simulink model "imfSILClaws"  (R2019a)
settings: Solver=FixedStepAuto  StartTime=0.0  StopTime=inf  FixedStep=.0125  RelTol=1e-3
libraries: etargetslib x2, dspnetwork x2, sldrtlib x1
settings Model: Creator=Chris  LastModifiedBy=Chris

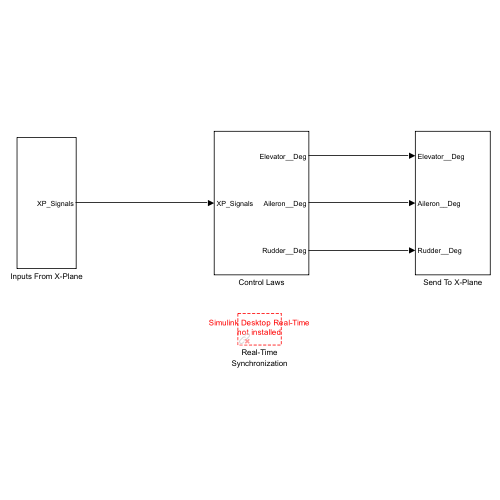
[thumbnail: Simulink's stored preview of the top-level diagram]
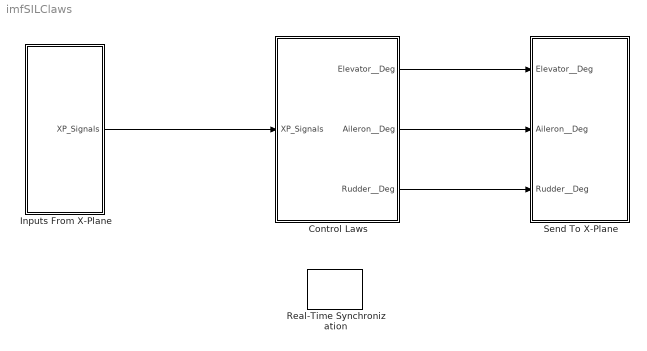
== system imfSILClaws ==
  Control Laws : Subsystem
  Inputs From X-Plane : Subsystem
  Real-Time Synchronization : sldrtlib/Real-Time Synchronization  SampleTime=.0125  MaxMissedTicks=10  ShowMissedTicks=off  YieldWhenWaiting=off
  Send To X-Plane : Subsystem
  wires:
  Inputs From X-Plane/1(XP_Signals) -> Control Laws/1(XP_Signals)
  Control Laws/1(Elevator__Deg) -> Send To X-Plane/1(Elevator__Deg)
  Control Laws/2(Aileron__Deg) -> Send To X-Plane/2(Aileron__Deg)
  Control Laws/3(Rudder__Deg) -> Send To X-Plane/3(Rudder__Deg)

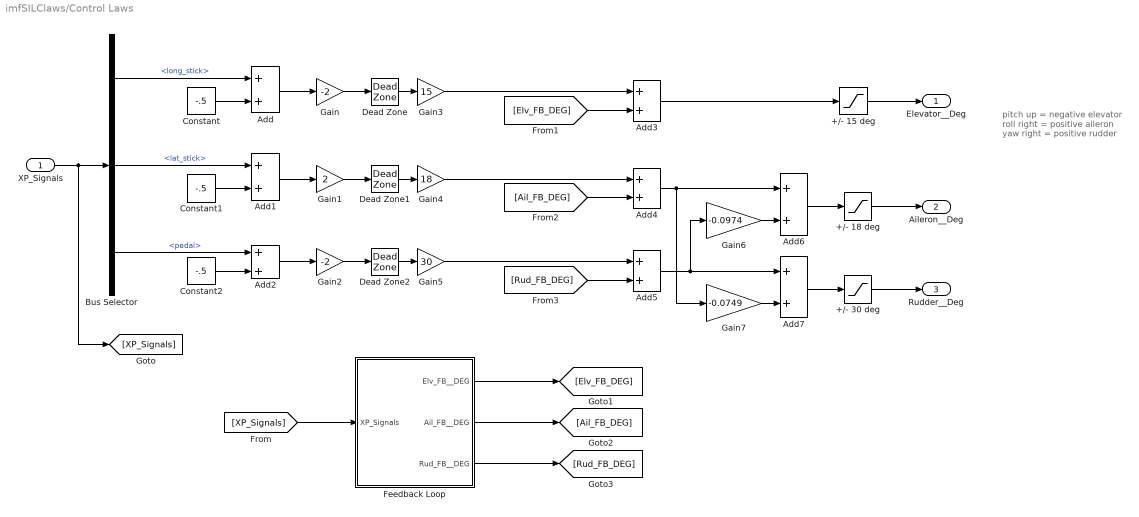
== system imfSILClaws/Control Laws ==
  note: pitch up = negative elevator
      | roll right = positive aileron
      | yaw right = positive rudder
  XP_Signals : Inport
  +/- 15 deg : Saturate  UpperLimit=15  LowerLimit=-15
  +/- 18 deg : Saturate  UpperLimit=18  LowerLimit=-18
  +/- 30 deg : Saturate  UpperLimit=30  LowerLimit=-30
  Add{,1..7} (8 alike) : Sum
  Bus Selector : BusSelector  OutputSignals=long_stick,lat_stick,pedal
  Constant : Constant  Value=-.5  OutDataTypeStr=single
  Constant1 : Constant  Value=-.5  OutDataTypeStr=single
  Constant2 : Constant  Value=-.5  OutDataTypeStr=single
  Dead Zone : DeadZone  LowerValue=-0.05  UpperValue=0.05  SaturateOnIntegerOverflow=on
  Dead Zone1 : DeadZone  LowerValue=-0.05  UpperValue=0.05  SaturateOnIntegerOverflow=on
  Dead Zone2 : DeadZone  LowerValue=-0.05  UpperValue=0.05  SaturateOnIntegerOverflow=on
  Feedback Loop : Subsystem
  Gain : Gain  Gain=-2
  Gain1 : Gain  Gain=2
  Gain2 : Gain  Gain=-2
  Gain3 : Gain  Gain=15
  Gain4 : Gain  Gain=18
  Gain5 : Gain  Gain=30
  Gain6 : Gain  Gain=-0.0974
  Gain7 : Gain  Gain=-0.0749
  Elevator__Deg : Outport
  Aileron__Deg : Outport  Port=2
  Rudder__Deg : Outport  Port=3
  wires:
  XP_Signals/1 -> [XP_Signals], Bus Selector/1
  +/- 18 deg/1 -> Aileron__Deg/1
  +/- 30 deg/1 -> Rudder__Deg/1
  +/- 15 deg/1 -> Elevator__Deg/1
  Bus Selector/1 -> Add/1  "<long_stick>"
  Bus Selector/3 -> Add2/1  "<pedal>"
  Constant/1 -> Add/2
  Constant1/1 -> Add1/2
  Bus Selector/2 -> Add1/1  "<lat_stick>"
  Constant2/1 -> Add2/2
  Add/1 -> Gain/1
  Add1/1 -> Gain1/1
  Add2/1 -> Gain2/1
  Gain1/1 -> Dead Zone1/1
  Gain2/1 -> Dead Zone2/1
  Gain3/1 -> Add3/1
  Gain4/1 -> Add4/1
  [XP_Signals] -> Feedback Loop/1(XP_Signals)
  Dead Zone/1 -> Gain3/1
  Dead Zone1/1 -> Gain4/1
  Dead Zone2/1 -> Gain5/1
  Add3/1 -> +/- 15 deg/1
  Add4/1 -> Add6/1, Gain7/1
  Add5/1 -> Add7/1, Gain6/1
  Gain/1 -> Dead Zone/1
  Feedback Loop/1(Elv_FB__DEG) -> [Elv_FB_DEG]
  Feedback Loop/2(Ail_FB__DEG) -> [Ail_FB_DEG]
  Feedback Loop/3(Rud_FB__DEG) -> [Rud_FB_DEG]
  [Elv_FB_DEG] -> Add3/2
  Gain5/1 -> Add5/1
  [Rud_FB_DEG] -> Add5/2
  [Ail_FB_DEG] -> Add4/2
  Add6/1 -> +/- 18 deg/1
  Add7/1 -> +/- 30 deg/1
  Gain6/1 -> Add6/2
  Gain7/1 -> Add7/2

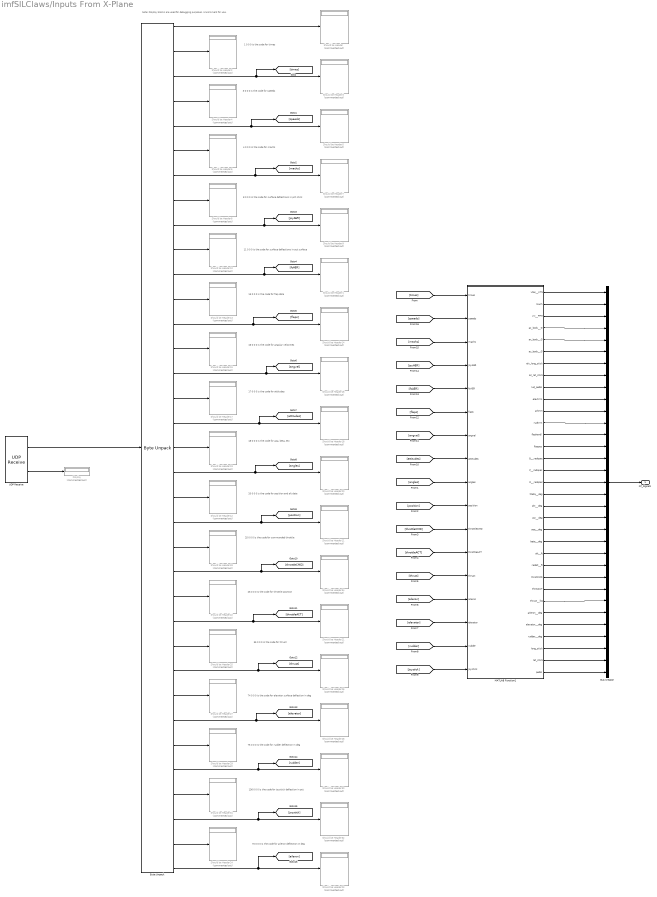
== system imfSILClaws/Inputs From X-Plane ==
  note: 26 0 0 0 is the code for throttle position
  note: 74 0 0 0 is the code for elevator surface deflection in deg
  note: 25 0 0 0 is the code for commanded throttle
  note: 75 0 0 0 is the code for rudder deflection in deg
  note: 13 0 0 0 is the code for flap data
  note: 17 0 0 0 is the code for attitudes
  note: 20 0 0 0 is the code for position and alt data
  note: 70 0 0 0 is the code for aileron deflection in deg
  note: 16 0 0 0 is the code for angular velocities
  note: 8 0 0 0 is the code for surface deflections in pct stick
  note: 3 0 0 0 is the code for speeds
  note: Note: Display blocks are used for debugging purposes. Uncomment for use.
  note: 4 0 0 0 is the code for machs
  note: 11 0 0 0 is the code for surface deflections in pct surface
  note: 136 0 0 0 is the code for joystick deflection in pct
  note: 1 0 0 0 is the code for times
  note: 35 0 0 0 is the code for thrust
  note: 18 0 0 0 is the code for aoa, beta, etc
  Bus Creator : BusCreator  Inputs=33
  Byte Unpack : etargetslib/Byte Unpack  dimensions={5,4,8,4,8,4,8,4,8,4,8,4,8,4,8,4,8,4,8,4,8,4,8,4,8,4,8,4,8,4,8,4,8,4,8}  datatypes={'uint8','uint8','single','uint8','single','uint8','single','uint8','single','uint8','single','uint8','single','uint8','single','uint8','single','uint8','single','uint8','single','uint8','single','uint8','single','uint8','single','uint8','single','uint8','single','uint8','single','uint8','single'}  byteAlign=1
  Display : Display  Commented=on
  MATLAB Function1 : MATLAB Function  TreatAsAtomicUnit=on
  Should be Header{,1..34} (35 alike) : Display  Commented=on
  UDP Receive : dspnetwork/UDP Receive  localURL='0.0.0.0'  localPort=45000  remoteURL='127.0.0.1'  remotePort=-1  recvBufferSize=8192  dims=617  signalDatatype=uint8  isComplex=off  isVarSize=off  showBlockingTime=off  blockingTime=0  sampletime=inf  blockPlatform=[]
  XP_Signals : Outport
  wires:
  Bus Creator/1 -> XP_Signals/1
  Byte Unpack/32 -> Should be Header31/1
  Byte Unpack/26 -> Should be Header25/1
  Byte Unpack/2 -> Should be Header2/1
  Byte Unpack/33 -> [joystick], Should be Header32/1
  MATLAB Function1/5(ax_body__G) -> Bus Creator/5
  Byte Unpack/21 -> [position], Should be Header11/1
  MATLAB Function1/8(ail_lat_stick) -> Bus Creator/8
  Byte Unpack/34 -> Should be Header24/1
  MATLAB Function1/22(beta__deg) -> Bus Creator/22
  Byte Unpack/11 -> [fcAER], Should be Header1/1
  Byte Unpack/23 -> [throttleCMD], Should be Header34/1
  MATLAB Function1/18(theta__deg) -> Bus Creator/18
  Byte Unpack/20 -> Should be Header12/1
  [throttleCMD] -> MATLAB Function1/11(throttleCMD)
  MATLAB Function1/21(aoa__deg) -> Bus Creator/21
  Byte Unpack/13 -> Should be Header14/1, [flaps]
  Byte Unpack/14 -> Should be Header15/1
  Byte Unpack/15 -> [angvel], Should be Header16/1
  [elevator] -> MATLAB Function1/15(elevator)
  [speeds] -> MATLAB Function1/2(speeds)
  Byte Unpack/17 -> [attitudes], Should be Header18/1
  [thrust] -> MATLAB Function1/13(thrust)
  MATLAB Function1/28(aileron__deg) -> Bus Creator/28
  MATLAB Function1/15(Q__radqsec) -> Bus Creator/15
  Byte Unpack/16 -> Should be Header17/1
  Byte Unpack/3 -> Should be Header3/1, [times]
  [flaps] -> MATLAB Function1/6(flaps)
  MATLAB Function1/13(flaphandl) -> Bus Creator/13
  MATLAB Function1/11(ailtrim) -> Bus Creator/11
  MATLAB Function1/29(elevator__deg) -> Bus Creator/29
  [angvel] -> MATLAB Function1/7(angvel)
  [position] -> MATLAB Function1/10(position)
  MATLAB Function1/12(rudtrim) -> Bus Creator/12
  MATLAB Function1/2(mach) -> Bus Creator/2
  MATLAB Function1/26(throtACT) -> Bus Creator/26
  MATLAB Function1/19(phi__deg) -> Bus Creator/19
  MATLAB Function1/17(R__radqsec) -> Bus Creator/17
  MATLAB Function1/24(radalt__ft) -> Bus Creator/24
  MATLAB Function1/7(elv_long_stick) -> Bus Creator/7
  MATLAB Function1/32(lat_stick) -> Bus Creator/32
  Byte Unpack/30 -> Should be Header29/1
  Byte Unpack/25 -> [throttleACT], Should be Header21/1
  MATLAB Function1/14(flappos) -> Bus Creator/14
  [joystick] -> MATLAB Function1/17(joystick)
  MATLAB Function1/33(pedal) -> Bus Creator/33
  MATLAB Function1/16(P__radqsec) -> Bus Creator/16
  Byte Unpack/6 -> Should be Header6/1
  Byte Unpack/18 -> Should be Header19/1
  Byte Unpack/28 -> Should be Header27/1
  Byte Unpack/7 -> [machs], Should be Header7/1
  Byte Unpack/1 -> Should be Header/1
  MATLAB Function1/23(alt__ft) -> Bus Creator/23
  MATLAB Function1/3(vvi__FPM) -> Bus Creator/3
  MATLAB Function1/30(rudder__deg) -> Bus Creator/30
  MATLAB Function1/6(ay_body__G) -> Bus Creator/6
  Byte Unpack/12 -> Should be Header13/1
  MATLAB Function1/9(rud_pedal) -> Bus Creator/9
  UDP Receive/2 -> Display/1
  UDP Receive/1 -> Byte Unpack/1
  [angles] -> MATLAB Function1/9(angles)
  [throttleACT] -> MATLAB Function1/12(throttleACT)
  [rudder] -> MATLAB Function1/16(rudder)
  Byte Unpack/5 -> [speeds], Should be Header5/1
  MATLAB Function1/10(elevtrim) -> Bus Creator/10
  Byte Unpack/29 -> [elevator], Should be Header28/1
  MATLAB Function1/20(psi__deg) -> Bus Creator/20
  [times] -> MATLAB Function1/1(times)
  Byte Unpack/4 -> Should be Header4/1
  Byte Unpack/24 -> Should be Header22/1
  Byte Unpack/8 -> Should be Header8/1
  Byte Unpack/9 -> [joyAER], Should be Header9/1
  Byte Unpack/27 -> [thrust], Should be Header26/1
  Byte Unpack/19 -> [angles], Should be Header20/1
  [attitudes] -> MATLAB Function1/8(attitudes)
  MATLAB Function1/4(az_body__G) -> Bus Creator/4
  MATLAB Function1/27(thrust__lbs) -> Bus Creator/27
  [aileron] -> MATLAB Function1/14(aileron)
  [joyAER] -> MATLAB Function1/4(joyAER)
  MATLAB Function1/25(throtCMD) -> Bus Creator/25
  Byte Unpack/35 -> [aileron], Should be Header23/1
  Byte Unpack/22 -> Should be Header33/1
  MATLAB Function1/1(vtas__KTS) -> Bus Creator/1
  MATLAB Function1/31(long_stick) -> Bus Creator/31
  [machs] -> MATLAB Function1/3(machs)
  Byte Unpack/10 -> Should be Header10/1
  Byte Unpack/31 -> [rudder], Should be Header30/1
  [fcAER] -> MATLAB Function1/5(fcAER)

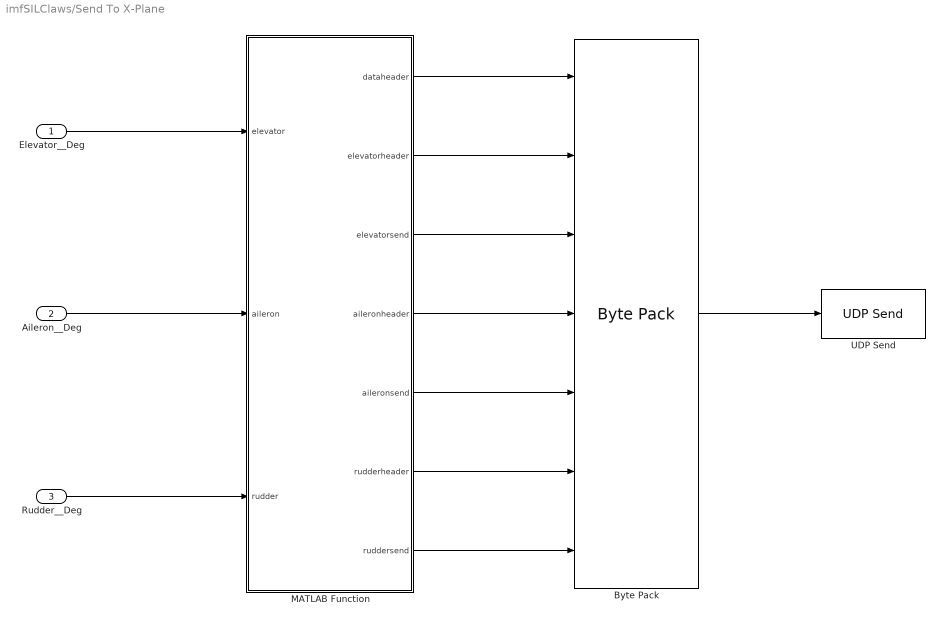
== system imfSILClaws/Send To X-Plane ==
  Elevator__Deg : Inport  OutDataTypeStr=single
  Aileron__Deg : Inport  Port=2  OutDataTypeStr=single
  Rudder__Deg : Inport  Port=3  OutDataTypeStr=single
  Byte Pack : etargetslib/Byte Pack  datatypes={'uint8', 'uint8', 'single', 'uint8', 'single','uint8', 'single'}  byteAlign=1
  MATLAB Function : MATLAB Function  TreatAsAtomicUnit=on
  UDP Send : dspnetwork/UDP Send  remoteURL='127.0.0.1'  remotePort=49000  localURL='0.0.0.0'  localPortSource=Automatically determine  localPort=-1  sampletime=-1  blockPlatform=[]  separateLengthPort=0
  wires:
  MATLAB Function/1(dataheader) -> Byte Pack/1
  MATLAB Function/7(ruddersend) -> Byte Pack/7
  Rudder__Deg/1 -> MATLAB Function/3(rudder)
  Elevator__Deg/1 -> MATLAB Function/1(elevator)
  MATLAB Function/3(elevatorsend) -> Byte Pack/3
  MATLAB Function/2(elevatorheader) -> Byte Pack/2
  MATLAB Function/5(aileronsend) -> Byte Pack/5
  Aileron__Deg/1 -> MATLAB Function/2(aileron)
  MATLAB Function/4(aileronheader) -> Byte Pack/4
  MATLAB Function/6(rudderheader) -> Byte Pack/6
  Byte Pack/1 -> UDP Send/1

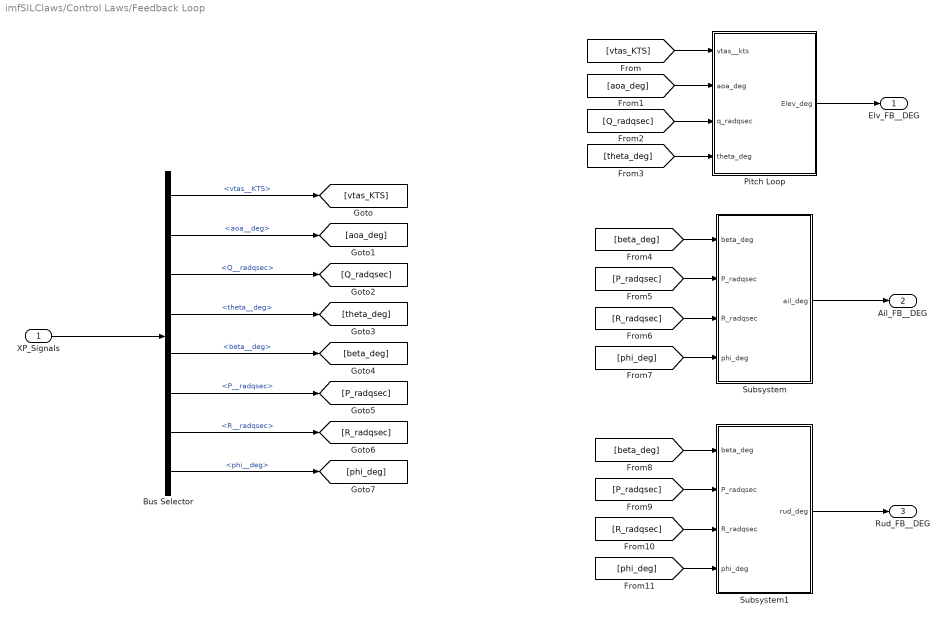
== system imfSILClaws/Control Laws/Feedback Loop ==
  XP_Signals : Inport
  Bus Selector : BusSelector  OutputSignals=vtas__KTS,aoa__deg,Q__radqsec,theta__deg,beta__deg,P__radqsec,R__radqsec,phi__deg
  Pitch Loop : Subsystem
  Subsystem : Subsystem
  Subsystem1 : Subsystem
  Elv_FB__DEG : Outport
  Ail_FB__DEG : Outport  Port=2
  Rud_FB__DEG : Outport  Port=3
  wires:
  XP_Signals/1 -> Bus Selector/1
  Bus Selector/1 -> [vtas_KTS]  "<vtas__KTS>"
  Bus Selector/2 -> [aoa_deg]  "<aoa__deg>"
  Bus Selector/3 -> [Q_radqsec]  "<Q__radqsec>"
  Bus Selector/4 -> [theta_deg]  "<theta__deg>"
  Bus Selector/5 -> [beta_deg]  "<beta__deg>"
  Bus Selector/6 -> [P_radqsec]  "<P__radqsec>"
  Bus Selector/7 -> [R_radqsec]  "<R__radqsec>"
  Bus Selector/8 -> [phi_deg]  "<phi__deg>"
  [vtas_KTS] -> Pitch Loop/1(vtas__kts)
  [aoa_deg] -> Pitch Loop/2(aoa_deg)
  [Q_radqsec] -> Pitch Loop/3(q_radqsec)
  [theta_deg] -> Pitch Loop/4(theta_deg)
  Pitch Loop/1(Elev_deg) -> Elv_FB__DEG/1
  [beta_deg] -> Subsystem/1(beta_deg)
  [P_radqsec] -> Subsystem/2(P_radqsec)
  [R_radqsec] -> Subsystem/3(R_radqsec)
  [phi_deg] -> Subsystem/4(phi_deg)
  [phi_deg] -> Subsystem1/4(phi_deg)
  [P_radqsec] -> Subsystem1/2(P_radqsec)
  [R_radqsec] -> Subsystem1/3(R_radqsec)
  [beta_deg] -> Subsystem1/1(beta_deg)
  Subsystem/1(ail_deg) -> Ail_FB__DEG/1
  Subsystem1/1(rud_deg) -> Rud_FB__DEG/1

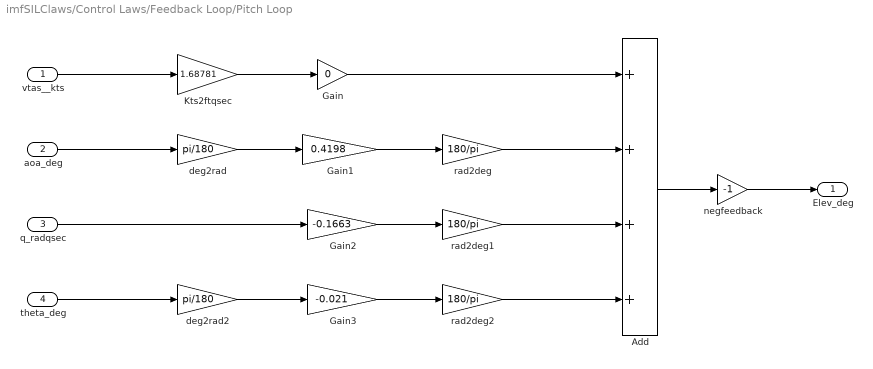
== system imfSILClaws/Control Laws/Feedback Loop/Pitch Loop ==
  vtas__kts : Inport
  aoa_deg : Inport  Port=2
  q_radqsec : Inport  Port=3
  theta_deg : Inport  Port=4
  Add : Sum  Inputs=++++
  Gain : Gain  Gain=0
  Gain1 : Gain  Gain=0.4198
  Gain2 : Gain  Gain=-0.1663
  Gain3 : Gain  Gain=-0.021
  Kts2ftqsec : Gain  Gain=1.68781
  deg2rad : Gain  Gain=pi/180
  deg2rad2 : Gain  Gain=pi/180
  negfeedback : Gain  Gain=-1
  rad2deg : Gain  Gain=180/pi
  rad2deg1 : Gain  Gain=180/pi
  rad2deg2 : Gain  Gain=180/pi
  Elev_deg : Outport
  wires:
  vtas__kts/1 -> Kts2ftqsec/1
  Kts2ftqsec/1 -> Gain/1
  aoa_deg/1 -> deg2rad/1
  deg2rad/1 -> Gain1/1
  Gain1/1 -> rad2deg/1
  Gain2/1 -> rad2deg1/1
  q_radqsec/1 -> Gain2/1
  Gain3/1 -> rad2deg2/1
  deg2rad2/1 -> Gain3/1
  theta_deg/1 -> deg2rad2/1
  rad2deg2/1 -> Add/4
  rad2deg/1 -> Add/2
  rad2deg1/1 -> Add/3
  Gain/1 -> Add/1
  Add/1 -> negfeedback/1
  negfeedback/1 -> Elev_deg/1

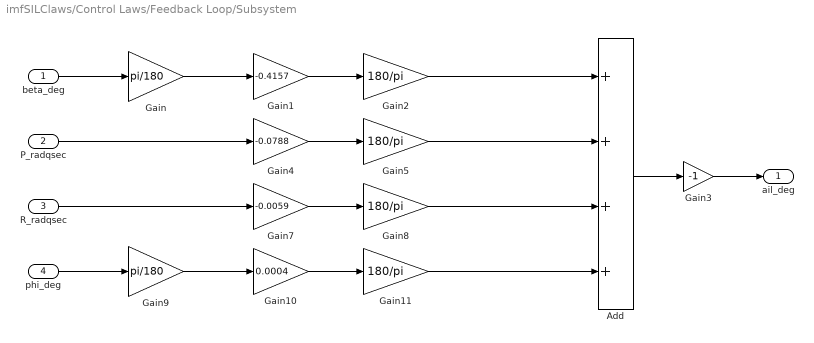
== system imfSILClaws/Control Laws/Feedback Loop/Subsystem ==
  beta_deg : Inport
  P_radqsec : Inport  Port=2
  R_radqsec : Inport  Port=3
  phi_deg : Inport  Port=4
  Add : Sum  Inputs=++++
  Gain : Gain  Gain=pi/180
  Gain1 : Gain  Gain=-0.4157
  Gain10 : Gain  Gain=0.0004
  Gain{2,5,8,11} (4 alike) : Gain  Gain=180/pi
  Gain3 : Gain  Gain=-1
  Gain4 : Gain  Gain=-0.0788
  Gain7 : Gain  Gain=-0.0059
  Gain9 : Gain  Gain=pi/180
  ail_deg : Outport
  wires:
  beta_deg/1 -> Gain/1
  Gain/1 -> Gain1/1
  Gain1/1 -> Gain2/1
  Gain4/1 -> Gain5/1
  P_radqsec/1 -> Gain4/1
  Gain7/1 -> Gain8/1
  R_radqsec/1 -> Gain7/1
  Gain10/1 -> Gain11/1
  Gain9/1 -> Gain10/1
  phi_deg/1 -> Gain9/1
  Gain2/1 -> Add/1
  Gain5/1 -> Add/2
  Gain8/1 -> Add/3
  Gain11/1 -> Add/4
  Add/1 -> Gain3/1
  Gain3/1 -> ail_deg/1

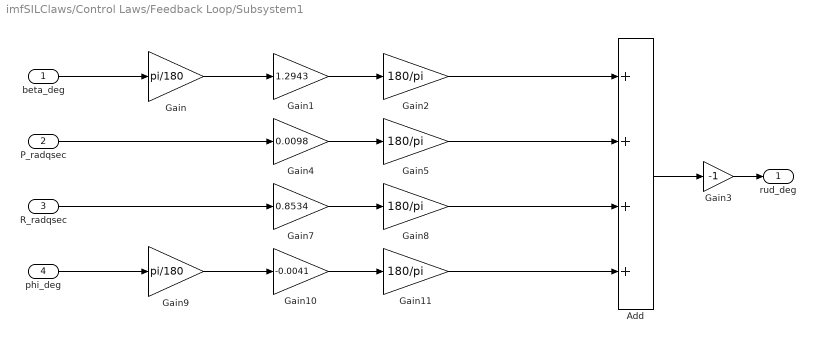
== system imfSILClaws/Control Laws/Feedback Loop/Subsystem1 ==
  beta_deg : Inport
  P_radqsec : Inport  Port=2
  R_radqsec : Inport  Port=3
  phi_deg : Inport  Port=4
  Add : Sum  Inputs=++++
  Gain : Gain  Gain=pi/180
  Gain1 : Gain  Gain=1.2943
  Gain10 : Gain  Gain=-0.0041
  Gain{2,5,8,11} (4 alike) : Gain  Gain=180/pi
  Gain3 : Gain  Gain=-1
  Gain4 : Gain  Gain=0.0098
  Gain7 : Gain  Gain=0.8534
  Gain9 : Gain  Gain=pi/180
  rud_deg : Outport
  wires:
  Gain1/1 -> Gain2/1
  Gain7/1 -> Gain8/1
  Gain8/1 -> Add/3
  Gain11/1 -> Add/4
  Gain5/1 -> Add/2
  Gain2/1 -> Add/1
  Gain/1 -> Gain1/1
  Gain4/1 -> Gain5/1
  Gain9/1 -> Gain10/1
  P_radqsec/1 -> Gain4/1
  R_radqsec/1 -> Gain7/1
  Add/1 -> Gain3/1
  Gain10/1 -> Gain11/1
  Gain3/1 -> rud_deg/1
  beta_deg/1 -> Gain/1
  phi_deg/1 -> Gain9/1

== matlab function imfSILClaws/Inputs From X-Plane/MATLAB Function1 ==
  data: times input; speeds input; machs input; joyAER input; fcAER input; flaps input; angvel input; attitudes input; angles input; position input; throttleCMD input; throttleACT input; thrust input; aileron input; elevator input; rudder input; joystick input; vtas__KTS output; mach output; vvi__FPM output; az_body__G output; ax_body__G output; ay_body__G output; elv_long_stick output; ail_lat_stick output; rud_pedal output; elevtrim output; ailtrim output; rudtrim output; flaphandl output; flappos output; Q__radqsec output; P__radqsec output; R__radqsec output; theta__deg output; phi__deg output; psi__deg output; aoa__deg output; beta__deg output; alt__ft output; radalt__ft output; throtCMD output; throtACT output; thrust__lbs output; aileron__deg output; elevator__deg output; rudder__deg output; long_stick output; lat_stick output; pedal output
function [vtas__KTS,mach,vvi__FPM,az_body__G,ax_body__G,ay_body__G,elv_long_stick,ail_lat_stick,rud_pedal,elevtrim, ailtrim, ...
          rudtrim,flaphandl,flappos,Q__radqsec,P__radqsec,R__radqsec,theta__deg,phi__deg,psi__deg,aoa__deg,beta__deg,alt__ft, ...
          radalt__ft,throtCMD,throtACT,thrust__lbs,aileron__deg,elevator__deg,rudder__deg,long_stick,lat_stick,pedal ] = ...
          fcn(times,speeds,machs,joyAER,fcAER,flaps,angvel,attitudes,angles,position,throttleCMD,throttleACT,thrust,aileron,elevator,rudder,joystick)

vtas__KTS       = speeds(3);
mach            = machs(1);
vvi__FPM        = machs(3);
az_body__G      = machs(5);
ax_body__G      = machs(6);
ay_body__G      = machs(7);
elv_long_stick  = joyAER(1);
ail_lat_stick   = joyAER(2);
rud_pedal       = joyAER(3);
elevtrim        = flaps(1);
ailtrim         = flaps(2);
rudtrim         = flaps(3);
flaphandl       = flaps(4);
flappos         = flaps(5);
Q__radqsec      = angvel(1);
P__radqsec      = angvel(2);
R__radqsec      = angvel(3);
theta__deg      = attitudes(1);
phi__deg        = attitudes(2);
psi__deg        = attitudes(3);
aoa__deg        = angles(1);
beta__deg       = angles(2);
alt__ft         = position(3);
radalt__ft      = position(4);
throtCMD     = throttleCMD(1);
throtACT     = throttleACT(1);
thrust__lbs     = thrust(1);
aileron__deg    = aileron(1); %roll right = positive
elevator__deg   = elevator(1); %pitch down = positive
rudder__deg     = rudder(1); %yaw right = positive
long_stick      = joystick(1); %full pitch down = 0, full pitch up =1
lat_stick       = joystick(2); %full roll left = 0, full roll right =1
pedal           = joystick(5); %full yaw right = 0, full yaw left =1
time = times;
fcsurf = fcAER;

== matlab function imfSILClaws/Send To X-Plane/MATLAB Function ==
  data: elevator input; dataheader output; aileron input; rudder input; elevatorheader output; elevatorsend output; aileronheader output; aileronsend output; rudderheader output; ruddersend output
function [dataheader, elevatorheader, elevatorsend, aileronheader, aileronsend, rudderheader, ruddersend] = fcn(elevator, aileron, rudder)

xpnull = single(-999); % X-Plane ignores -999
dataheader =[uint8(68) uint8(65) uint8(84) uint8(65) uint8(0)];
elevatorheader = [uint8(74) uint8(0) uint8(0) uint8(0)];
aileronheader = [uint8(70) uint8(0) uint8(0) uint8(0)];
rudderheader = [uint8(75) uint8(0) uint8(0) uint8(0)];
elevatorsend = [single(elevator) single(elevator) single(elevator) single(elevator) xpnull xpnull xpnull xpnull];
ruddersend = [single(rudder) xpnull single(rudder) xpnull xpnull xpnull xpnull xpnull];
aileronsend = [single(aileron) -single(aileron) xpnull xpnull xpnull xpnull xpnull xpnull];
